simulink model "Izhikevich_QIF"  (R2019a)
settings: Solver=VariableStepAuto  StartTime=0.0  StopTime=1000  RelTol=1e-9
values from neighbouring files (symbols this model uses):
  c = -50    [H_H_Mod.m]    (also in Part2.m = -65)
  d = 2    [H_H_Mod.m]    (also in Part2.m = 8)
undefined symbols (not defined in the file or in its folder): sigbuilder_block
libraries: simulink x1
settings Model: Creator=Pranav Maddula  LastModifiedBy=Pranav Maddula

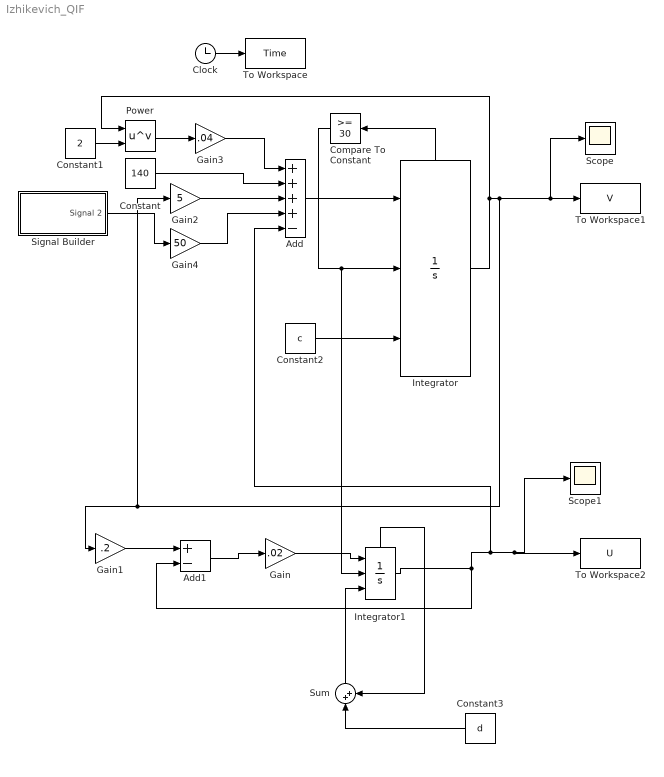
== system Izhikevich_QIF ==
  Add : Sum  Inputs=++++-
  Add1 : Sum  Inputs=+-
  Clock : Clock
  Compare To Constant : simulink/Logic and Bit Operations/Compare To Constant  relop=>=  const=30  OutDataTypeStr=boolean
  Constant : Constant  Value=140
  Constant1 : Constant  Value=2
  Constant2 : Constant  Value=c
  Constant3 : Constant  Value=d
  Gain : Gain  Gain=.02
  Gain1 : Gain  Gain=.2
  Gain2 : Gain  Gain=5
  Gain3 : Gain  Gain=.04
  Gain4 : Gain  Gain=50
  Integrator : Integrator  ExternalReset=either  InitialConditionSource=external  LimitOutput=on  UpperSaturationLimit=30  LowerSaturationLimit=-80  ShowStatePort=on
  Integrator1 : Integrator  ExternalReset=either  InitialConditionSource=external  WrappedStateUpperValue=100  WrappedStateLowerValue=0  ShowStatePort=on  IgnoreLimit=on
  Power : Math  Operator=pow  SaturateOnIntegerOverflow=on
  Scope : Scope
  Scope1 : Scope
  Signal Builder : Subsystem  Tag=STV Subsys  LoadFcn=sigbuilder_block('load');  StartFcn=sigbuilder_block('start');  StopFcn=sigbuilder_block('stop');  ClipboardFcn=sigbuilder_block('clipboard');  mask(Sigbuilder block){tuvar=[0:10]}
      mask help: Simulink:masks:SigbuilderBlock_MD
      mask init:
      | if ~strcmp(get_param(bdroot(gcbh),'SimulationStatus'),'stopped') tuvar = sigbuilder_block('maskInit'); end
      settings: CopyFcn=sigbuilder_block('copy');  DeleteFcn=sigbuilder_block('delete');  ModelCloseFcn=sigbuilder_block('modelClose');  PreSaveFcn=sigbuilder_block('preSave');  PauseFcn=sigbuilder_block('pause');  ContinueFcn=sigbuilder_block('continue');  NameChangeFcn=sigbuilder_block('namechange');  OpenFcn=sigbuilder_block('open',[437.6 199.2 550.4 400 ]);  CloseFcn=sigbuilder_block('close');
      mask Display: plot(0, 0, 100, 100,[2, 2, 32, 32, 2], [68, 8, 8, 68, 68],[32, 2], [38, 38], [32, 19, 2],[53, 60, 44], [32, 17, 17, 2],[16, 16, 31, 31]);txt = getActiveGroup(gcbh);text(2, 100, txt,'verticalAlignment', 'top');
  Sum : Sum  Inputs=|++
  To Workspace : ToWorkspace  VariableName=Time  SampleTime=-1
  To Workspace1 : ToWorkspace  VariableName=V  SampleTime=-1
  To Workspace2 : ToWorkspace  VariableName=U  SampleTime=-1
  wires:
  Add/1 -> Integrator/1
  Gain/1 -> Integrator1/1
  Add1/1 -> Gain/1
  Gain1/1 -> Add1/1
  Integrator/1 -> Power/1, Scope/1, To Workspace1/1, Gain2/1, Gain1/1
  Gain2/1 -> Add/3
  Constant/1 -> Add/2
  Constant1/1 -> Power/2
  Power/1 -> Gain3/1
  Gain3/1 -> Add/1
  Clock/1 -> To Workspace/1
  Constant2/1 -> Integrator/3
  Compare To Constant/1 -> Integrator1/2, Integrator/2
  Integrator/State -> Compare To Constant/1
  Gain4/1 -> Add/4
  Signal Builder/1(Signal 2) -> Gain4/1
  Integrator1/1 -> To Workspace2/1, Scope1/1, Add/5, Add1/2
  Constant3/1 -> Sum/1
  Sum/1 -> Integrator1/3
  Integrator1/State -> Sum/2

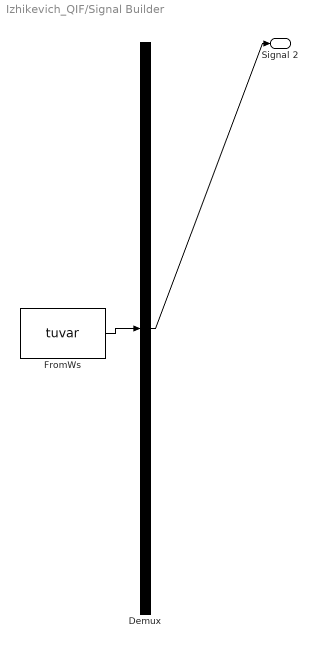
== system Izhikevich_QIF/Signal Builder ==
  Demux : Demux  Tag=STV Demux  Outputs=1
  FromWs : FromWorkspace  Tag=STV FromWs  VariableName=tuvar  SampleTime=0
      SigBuilderData=|
      | common.afterFinalStr = 'Extrapolate'
      | common.sampleTime = 0
      | dataSet.timeRange = [0 1000]
      | dataSet.name = 'Group 1'
      | sbobj.Groups.Name = 'Group 1'
      | sbobj.Groups.Signals.Name = 'Signal 2'
      | sbobj.Groups.Signals.XData = [0 5 15 600 1000]
      | sbobj.Groups.Signals.YData = [0 0 1 1 1]
      | sbobj.Groups.TimeRange = [0 1000]
  Signal 2 : Outport  Tag=STV Outport
  wires:
  FromWs/1 -> Demux/1
  Demux/1 -> Signal 2/1
